simulink model "PEC11R"  (R2024b)
settings: Solver=FixedStepAuto  StartTime=0.0  StopTime=10  FixedStep=0.1  RelTol=1e-3  EnableMultiTasking=on
libraries: stm32f4xxblockslib x3, stm32g4xxblockslib x3, simulink x1
settings Model: STM32="{\"DigitalPortRead\":[{\"ID\":\"e:8\"},{\"ID\":\"e:9\"},{\"ID\":\"e:38\"},{\"ID\":\"e:39\"},{\"ID\":\"PEC11R:38\"},{\"ID\":\"PEC11R:9\"},{\"ID\":\"PEC11R:8\"}],\"EncoderBlockForG4\":[{\"ID\":\"e:26\"},{\"ID\":\"e:27\"},{\"ID\":\"e:28\"}]}"  SimulationMode=external  Creator=gamen  LastModifiedBy=gamen
settings OptimizationCC: DefaultParameterBehavior=Inlined  EnhancedBackFolding=on  PassReuseOutputArgsAs=Individual arguments  ZeroExternalMemoryAtStartup=off  ZeroInternalMemoryAtStartup=off  MaxStackSize=512  OptimizeBlockOrder=speed  DifferentSizesBufferReuse=on  OptimizationCustomize=off  EfficientTunableParamExpr=on
settings DebuggingCC: ParameterTunabilityLossMsg=error
settings HardwareCC: ProdBitPerPointer=32  ProdBitPerSizeT=32  ProdBitPerPtrDiffT=32  ProdLargestAtomicInteger=Long  ProdLargestAtomicFloat=Double  ProdWordSize=32  ProdLongLongMode=on  ProdHWDeviceType=ARM Compatible->ARM Cortex-M
settings SFSimCC: MATLABDynamicMemAlloc=off
settings RTWCC: Description=Embedded Coder  SystemTargetFile=ert.tlc  HardwareBoard=STM32G4xx Based  TemplateMakefile=ert_default_tmf  Toolchain=GNU Tools for ARM Embedded Processors
settings CodeAppCC: ForceParamTrailComments=on  IgnoreCustomStorageClasses=off  OperatorAnnotations=on  SimulinkDataObjDesc=on  SFDataObjDesc=on  InsertBlockDesc=on
settings ERTTargetCC: TargetLangStandard=C99 (ISO)  CodeReplacementLibrary=ARM Cortex-M  ExtModeTransport=3  ExtModeStaticAlloc=on  ExtModeStaticAllocSize=2048  ExtModeMexFile=ext_xcp  ExtModeIntrfLevel=Level2 - Open

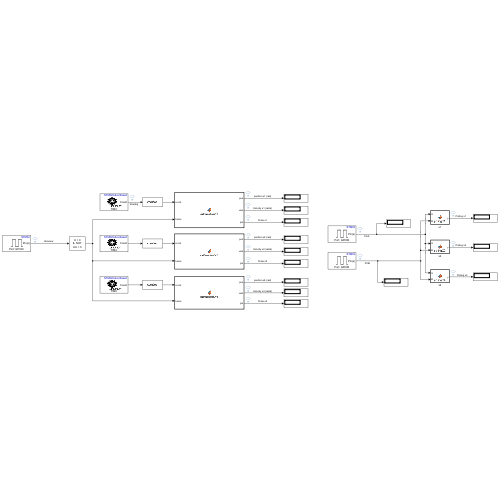
[thumbnail: Simulink's stored preview of the top-level diagram]
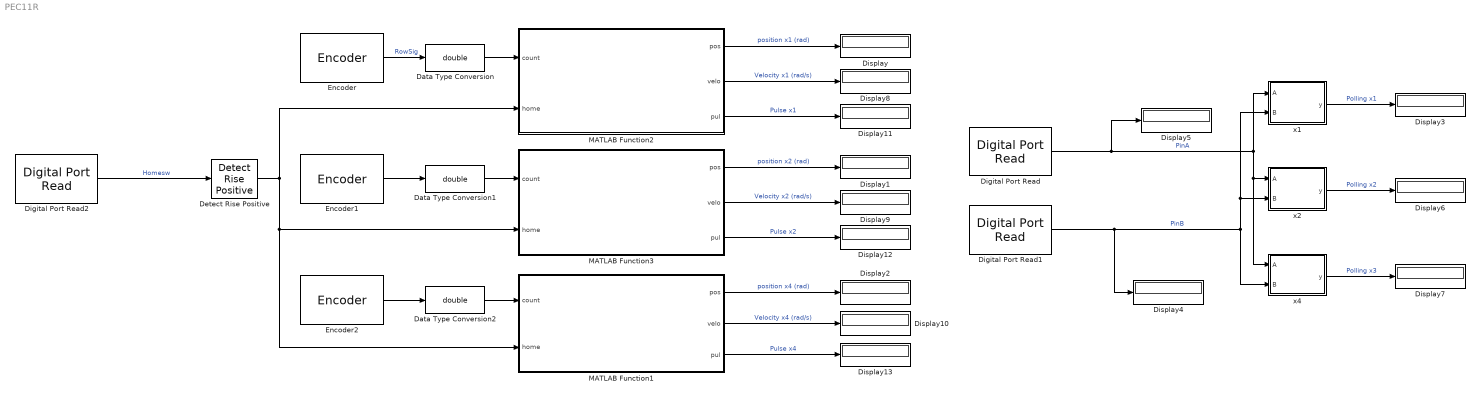
== system PEC11R ==
  Data Type Conversion : DataTypeConversion  OutDataTypeStr=double  SaturateOnIntegerOverflow=off  RndMeth=Floor
  Data Type Conversion1 : DataTypeConversion  OutDataTypeStr=double  SaturateOnIntegerOverflow=off  RndMeth=Floor
  Data Type Conversion2 : DataTypeConversion  OutDataTypeStr=double  SaturateOnIntegerOverflow=off  RndMeth=Floor
  Detect Rise Positive : simulink/Logic and Bit Operations/Detect Rise Positive  vinit=0  OutDataTypeStr=boolean
  Digital Port Read : stm32f4xxblockslib/Digital Port Read  PortName=GPIOB  PinNumber=[4]  ReadOperation=on  IOAsArray=on  SampleTime=-1  EnableSimPort=off  hoistedMaskSrc=ECSoC/ECSimCodegen/Digital Port Read
      settings: LibrarySourceBlock=stm32g4xxblockslib/Digital Port Read
  Digital Port Read1 : stm32f4xxblockslib/Digital Port Read  PortName=GPIOB  PinNumber=[5]  ReadOperation=on  IOAsArray=on  SampleTime=-1  EnableSimPort=off  hoistedMaskSrc=ECSoC/ECSimCodegen/Digital Port Read
      settings: LibrarySourceBlock=stm32g4xxblockslib/Digital Port Read
  Digital Port Read2 : stm32f4xxblockslib/Digital Port Read  PortName=GPIOC  PinNumber=[13]  ReadOperation=on  IOAsArray=on  SampleTime=-1  EnableSimPort=off  hoistedMaskSrc=ECSoC/ECSimCodegen/Digital Port Read
      settings: LibrarySourceBlock=stm32g4xxblockslib/Digital Port Read
  Display{,1..13} (14 alike) : Display
  Encoder : stm32g4xxblockslib/Encoder  TimerModule=TIM3  EnableResetInput=off  OutputCountAfterFirstIndex=off  OutputValidIndex=off  OutputDirection=off  OutputStatus=off  SampleTime=-1
  Encoder1 : stm32g4xxblockslib/Encoder  TimerModule=TIM4  EnableResetInput=off  OutputCountAfterFirstIndex=off  OutputValidIndex=off  OutputDirection=off  OutputStatus=off  SampleTime=-1
  Encoder2 : stm32g4xxblockslib/Encoder  TimerModule=TIM8  EnableResetInput=off  OutputCountAfterFirstIndex=off  OutputValidIndex=off  OutputDirection=off  OutputStatus=off  SampleTime=-1
  MATLAB Function1 : MATLAB Function  TreatAsAtomicUnit=on
  MATLAB Function2 : MATLAB Function  TreatAsAtomicUnit=on
  MATLAB Function3 : MATLAB Function  TreatAsAtomicUnit=on
  x1 : MATLAB Function  TreatAsAtomicUnit=on
  x2 : MATLAB Function  TreatAsAtomicUnit=on
  x4 : MATLAB Function  TreatAsAtomicUnit=on
  wires:
  MATLAB Function3/1(pos) -> Display1/1  "position x2 (rad)"
  Encoder2/1 -> Data Type Conversion2/1
  x2/1(y) -> Display6/1  "Polling x2"
  x4/1(y) -> Display7/1  "Polling x3"
  MATLAB Function2/1(pos) -> Display/1  "position x1 (rad)"
  MATLAB Function3/2(velo) -> Display9/1  "Velocity x2 (rad/s)"
  Data Type Conversion/1 -> MATLAB Function2/1(count)
  MATLAB Function1/3(pul) -> Display13/1  "Pulse x4"
  Encoder/1 -> Data Type Conversion/1  "RowSig"
  Data Type Conversion2/1 -> MATLAB Function1/1(count)
  Digital Port Read1/1 -> x1/2(B), x2/2(B), x4/2(B), Display4/1  "PinB"
  Data Type Conversion1/1 -> MATLAB Function3/1(count)
  MATLAB Function1/1(pos) -> Display2/1  "position x4 (rad)"
  MATLAB Function3/3(pul) -> Display12/1  "Pulse x2"
  Digital Port Read/1 -> Display5/1, x1/1(A), x4/1(A), x2/1(A)  "PinA"
  x1/1(y) -> Display3/1  "Polling x1"
  MATLAB Function2/2(velo) -> Display8/1  "Velocity x1 (rad/s)"
  MATLAB Function1/2(velo) -> Display10/1  "Velocity x4 (rad/s)"
  MATLAB Function2/3(pul) -> Display11/1  "Pulse x1"
  Encoder1/1 -> Data Type Conversion1/1
  Digital Port Read2/1 -> Detect Rise Positive/1  "Homesw"
  Detect Rise Positive/1 -> MATLAB Function3/2(home), MATLAB Function1/2(home), MATLAB Function2/2(home)

== matlab function PEC11R/x1 ==
  data: A input; y output; B input
function y =  pollingX1(A, B)
    persistent c stageA
    if isempty(c)
        c = 0;
        stageA = 1;
    end

    if A == 0 && stageA
        stageA = 0;
        c = c + 2 * B - 1;
    elseif A == 1
        stageA = 1;
    end

    y = c;
end

== matlab function PEC11R/MATLAB Function2 ==
  data: count input; pos output; velo output; pul output; home input
function [pos, velo, pul] = calFunctionX1(count, home)
    persistent pulse lastpulse lastrad home_position;
    
    if isempty(pulse)
        pulse = 0;
        lastpulse = 0;
        lastrad = 0;
        home_position = 0;
    end
    
    pulse_diff = count - lastpulse;
    if abs(pulse_diff) > 65520
        pulse = pulse + (65520 * sign(pulse_diff) - pulse_diff);
    else
        pulse = pulse + pulse_diff;
    end
    
    if home == 1
        home_position = pulse;
    end

    pul = pulse - home_position;
    pos = pul * (2 * pi / 24);
    velo = (pos - lastrad) / 0.1;
    
    lastpulse = count;
    lastrad = pos;
end

== matlab function PEC11R/MATLAB Function3 ==
  data: count input; pos output; velo output; pul output; home input
function [pos, velo, pul] = calFunctionX2(count, home)
    persistent pulse lastpulse lastrad home_position;
    
    if isempty(pulse)
        pulse = 0;
        lastpulse = 0;
        lastrad = 0;
        home_position = 0;
    end
    
    pulse_diff = count - lastpulse;
    if abs(pulse_diff) > 10000
        pulse = pulse + (65520 * sign(pulse_diff) - pulse_diff);
    else
        pulse = pulse + pulse_diff;
    end
    
    if home == 1
        home_position = pulse;
    end

    pul = pulse - home_position;
    pos = pul * (2 * pi / 48);
    velo = (pos - lastrad) / 0.1;
    
    lastpulse = count;
    lastrad = pos;
end

== matlab function PEC11R/MATLAB Function1 ==
  data: count input; pos output; velo output; pul output; home input
function [pos, velo, pul] = calFunctionX4(count, home)
    persistent pulse lastpulse lastrad home_position;
    
    if isempty(pulse)
        pulse = 0;
        lastpulse = 0;
        lastrad = 0;
        home_position = 0;
    end
    
    pulse_diff = count - lastpulse;
    if abs(pulse_diff) > 10000
        pulse = pulse + (65472 * sign(pulse_diff) - pulse_diff);
    else
        pulse = pulse + pulse_diff;
    end
    
    if home == 1
        home_position = pulse;
    end

    pul = pulse - home_position;
    pos = pul * (2 * pi / 96);
    velo = (pos - lastrad) / 0.1;
    
    lastpulse = count;
    lastrad = pos;
end

== matlab function PEC11R/x2 ==
  data: A input; y output; B input
function y = pollingX2(A, B)
    persistent c stageA
    if isempty(c)
        c = 0;
        stageA = 1;
    end

    if A == 0 && stageA
        stageA = 0;
        c = c + 2 * B - 1;
    elseif A == 1 && ~stageA
        stageA = 1;
        c = c + 1 - 2 * B;
    end

    y = c;
end

== matlab function PEC11R/x4 ==
  data: A input; y output; B input
function y = pollingX4(A, B)
    persistent c stageA stageB
    if isempty(c)
        c = 0;
        stageA = 1;
        stageB = 1;
    end

    if A == 0 && stageA
        stageA = 0;
        c = c + 2 * B - 1;
    elseif A == 1 && ~stageA
        stageA = 1;
        c = c + 1 - 2 * B;
    end

    if B == 0 && stageB
        stageB = 0;
        c = c + 2 * (A == 0) - 1;
    elseif B == 1 && ~stageB
        stageB = 1;
        c = c + 2 * (A == 1) - 1;
    end

    y = c;
end
